simulink model "second_block"  (R2022a)
settings: Solver=VariableStepAuto  StartTime=0.0  StopTime=10.0  RelTol=1e-3
libraries: simulink x2
settings Model: Creator=User  LastModifiedBy=User

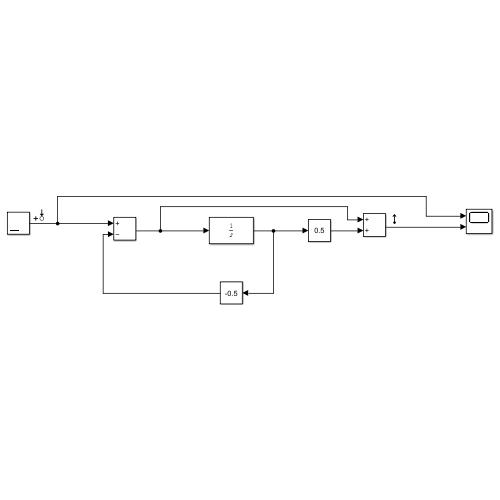
[thumbnail: Simulink's stored preview of the top-level diagram]
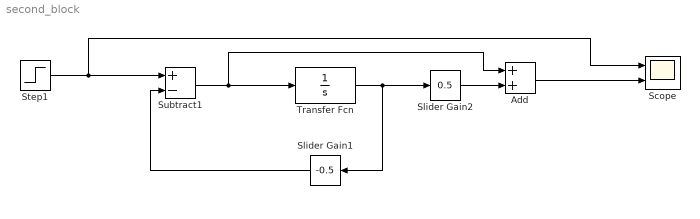
== system second_block ==
  Add : Sum
  Scope : Scope  NumInputPorts=2
  Slider Gain1 : simulink/Math Operations/Slider Gain  gain=-0.5  low=-1  high=2
  Slider Gain2 : simulink/Math Operations/Slider Gain  gain=0.5  low=-0.5  high=2
  Step1 : Step  SampleTime=0
  Subtract1 : Sum  Inputs=+-
  Transfer Fcn : TransferFcn  Numerator=1  Denominator=[1 0]
  wires:
  Subtract1/1 -> Add/1, Transfer Fcn/1
  Transfer Fcn/1 -> Slider Gain2/1, Slider Gain1/1
  Slider Gain1/1 -> Subtract1/2
  Step1/1 -> Scope/1, Subtract1/1
  Slider Gain2/1 -> Add/2
  Add/1 -> Scope/2
